simulink model "Linear_Approximation"  (R2019a)
settings: Solver=FixedStepDiscrete  StartTime=0.0  StopTime=t_end  RelTol=1e-3
InitFcn:
  | clear;
  | DIAGNOSTIC = 0;  %% flag to give more information as simulation proceeds such as comments & plots
  | CALIB_DIAGNOSTIC =  0; %% flag to give more information about calibration of filterbank due to overlap between filters: Mar 2016
  | PRESCRIPT = 1;  %% flag to plot requested versus achieved insertion gains (esp for 125-250 Hz region).
  | ipfiledigrms = -36; %% input file RMS in dB for 65 dB SPL equivalent
  | opfiledigrms = -36; %% output file RMS in dB for 65 dB SPL equivalent
  | equiv_ipSPL = 65; %% simulation of signal at this level through aid`
  | X_high = 1; % Maximum input
  | ref_dB = 85; X_ref = 1; % Define a reference point in X and its dBA value
  | re_level = 10.^(.05*(equiv_ipSPL-65)); %% scale factor at start of hearing aid, to get input to desired simulation level
  | M_bits = 5;   % decides length of tables, 2^(4+M_bits)
  | 
  | NChans = 5;
  | [chan_cfs, chan_thrs, t_atts, t_rels] ...
  |    = InitializeCompressionSettings(NChans);
  | % AidSettings5Chans;
  | 
  | %[VALID_WAV_FILE, sig, Fs, nbits, file_rms_dB, NStreams] ...
  | %  = loadwavfile(ipfiledigrms); %%  find [Fs], performs [recalculate] externally, provided valid file found
  | VALID_WAV_FILE = 1;
  | %[newfile, newpath] = uigetfile('*.wav','Open Signal File To Process.....');
  | %if isequal(newfile,0) || isequal(newpath,0)
  | %    fprintf(1,'\nFile not found'); VALID_WAV_FILE = 0;
  | %else
  | %    [sig, Fs] = audioread(strcat(newpath,newfile));
  | %end
  | X_thresh = 1*10^(0.05*(0-85));
  | 
  | Amplitudes = [X_thresh, X_thresh*10, X_thresh*100, X_thresh*1000, X_thresh*10000, 1]; %, X_thresh*100000];
  | 
  | fMin = 100; %Hz
  | fMax = 10000; %Hz
  | Fs = 48000; %Hz
  | Ts = 1/Fs;
  | %tt = (0:length(sig)-1 )./Fs;
  | tt = 0:Ts:4;
  | deltaF = (fMax - fMin)/tt(end);
  | X_sweep = Amplitudes'*sin(2*pi*(fMin*tt +  0.5*deltaF*tt.*tt)) ;
  | 
  | Fs = 48000;
  | Volume = 6;
  | sig = X_sweep(Volume,:)';
  | opplayer  = audioplayer(sig, Fs);
  | nbits = opplayer.bitspersample;
  | %sig = resample(sig,48000,Fs);
  | %Fs = 48000;
  | 
  | 
  | NStreams = min(size(sig));
  | EQ_SPAN_MSEC = 6;
  | 
  | insrt_frqs = [125, 250, 500, 1000, 2000, 3000, 4000, 6000, 8000, 10000 ]; %% decimal values
  | insrt_gns = [0 3 5 10 15 20 25 30 30 30]; %% prescribed dB for 65 dB input
  | %insrt_gns = 5*ones(1,length(insrt_frqs));  %no prescription
  | n_insrts = length(insrt_gns);
  | 
  | UPPER_FREQ_LIM = min(11e3, 0.90*Fs/2);
  | [ig_eq, calib_bpfs, dig_chan_lvl_0dBgain, dig_chan_dBthrs, Calib_recomb_dBpost] ...
  |     = update_channel_params(Fs, NChans, chan_cfs, chan_thrs, insrt_frqs, insrt_gns, ...
  |     0.1, UPPER_FREQ_LIM, EQ_SPAN_MSEC, PRESCRIPT, DIAGNOSTIC, CALIB_DIAGNOSTIC) ;  %% calculates channel edge frequencies, generates expected band levels for LTASS SWN to calibrate compressors & filterbank
  | 
  | recombGain = 10.^(0.05.*Calib_recomb_dBpost);
  | 
  | % translate sig into a form simulink likes
  | % Ts = 1/Fs;
  | % tt = (0:length(sig)-1).*Ts;
  | %t_end = tt(5*2^(M_bits+4) );   % to test table fill
  | t_end = tt(end);
  | sig_in = [tt', sig];
  | min_thresh_dB = 0;
  | for ix = 1:NChans
  |    [Gain_Table(:,ix), max_gain_prescript(ix), X_in(:,ix), chan_crs(ix)] ...
  |      = Compression_Wrapper_V2(Fs, min_thresh_dB, ...
  |      X_high, calib_bpfs(:,ix), ig_eq, ref_dB, X_ref, M_bits);
  | end
  | 
  | Initialize_Delay_Values;
  | Initialize_AGC_Consts;
  | W_bits = 32;
  | F_bits = 28;
  | M_bits = 5;
  | M_Bits = M_bits;
  | 
  | % Generating signals for simulink
  | Table_Fill = zeros(1,length(tt))';
  | Table_Fill(1                : 2^(M_bits+4) )  = Gain_Table(:,1);
  | Table_Fill(2^(M_bits+4)+1   : 2*2^(M_bits+4) )= Gain_Table(:,2);
  | Table_Fill(2*2^(M_bits+4)+1 : 3*2^(M_bits+4) )= Gain_Table(:,3);
  | Table_Fill(3*2^(M_bits+4)+1 : 4*2^(M_bits+4) )= Gain_Table(:,4);
  | Table_Fill(4*2^(M_bits+4)+1 : 5*2^(M_bits+4) )= Gain_Table(:,5);
  | Table_Fill = [tt', Table_Fill];
  | Fill_Valid = zeros(1,length(tt))';
  | Fill_Valid(1:5*2^(M_bits+4)) = 1;
  | Fill_Valid = boolean(Fill_Valid);
  | Fill_Valid = [tt', Fill_Valid];
  | t_att = t_atts./1000; s_att = t_att.*Fs; % change units of t_atts from ms to samples
  | t_rel = t_rels./1000; s_rel = t_rel.*Fs; % change units of t_rels from ms to samples
  | r_att = nthroot(0.1, s_att);
  | r_rel = nthroot(0.1, s_rel);
  | 
  | Reset = [tt', boolean(zeros(1,length(tt)))'];
StopFcn:
  | proc_sig = double(out.proc_sig.data(:));
  | %alignedSigs = double(out.alignedSigs.data(:));
  | [opwav, stop_ok] = savewavfile(opfiledigrms, ipfiledigrms, proc_sig, Fs, nbits, NStreams);
  | 
  | load('SweepSimOutput.mat')
  | X_out_Sweep_Sim(Volume,:) = proc_sig;
  | save('SweepSimOutput.mat', 'X_out_Sweep_Sim');
libraries: hdlsllib x33, simulink x2
settings Model: Creator=Bailey  LastModifiedBy=Bailey
settings DataIOCC: SaveOutput=off  SaveTime=off
settings OptimizationCC: BlockReduction=off  ConditionallyExecuteInputs=off  DefaultParameterBehavior=Inlined
settings DebuggingCC: AlgebraicLoopMsg=error  SingleTaskRateTransMsg=error
settings HardwareCC: ProdBitPerPointer=32  ProdBitPerSizeT=32  ProdBitPerPtrDiffT=32  ProdLargestAtomicFloat=None  ProdIntDivRoundTo=Undefined  ProdEndianess=Unspecified  ProdWordSize=32  ProdHWDeviceType=ASIC/FPGA->ASIC/FPGA  TargetBitPerPointer=64  TargetBitPerSizeT=64  TargetBitPerPtrDiffT=64  TargetLongLongMode=on  TargetIntDivRoundTo=Zero  TargetEndianess=LittleEndian  TargetWordSize=64  TargetHWDeviceType=Custom Processor->MATLAB Host Computer  ProdEqTarget=off

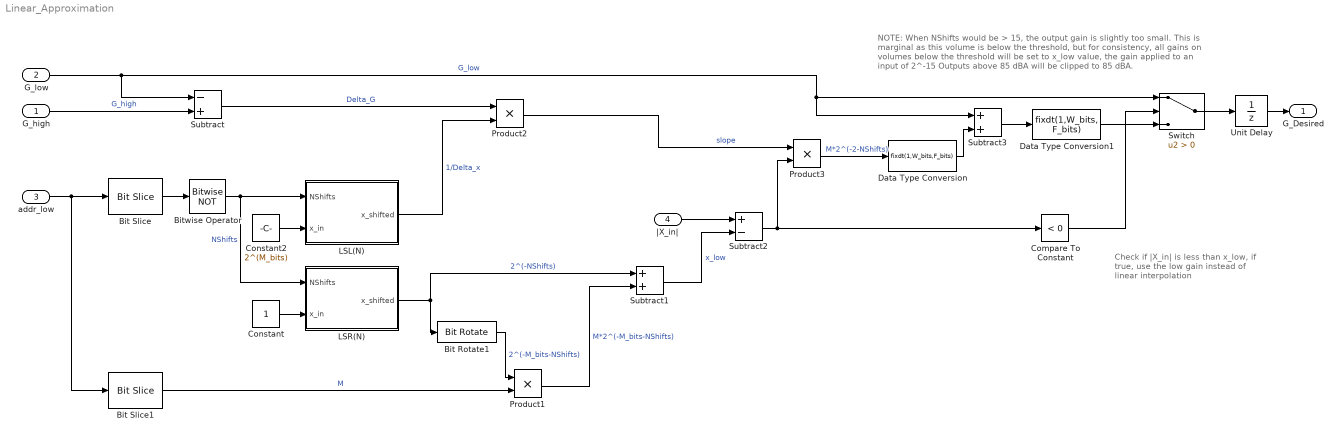
== system Linear_Approximation ==
  note: Check if |X_in| is less than x_low,
      | if true, use the low gain instead of
      | linear interpolation
  note: NOTE: When NShifts would be > 15, the output gain is slightly too small.
      | This is marginal as this volume is below the threshold, but for consistency,
      | all gains on volumes below the threshold will be set to x_low value, the
      | gain applied to an input of 2^-15
      | Outputs above 85 dBA will be clipped to 85 dBA.
  G_high : Inport  OutDataTypeStr=fixdt(1,32,28)  PortDimensions=1  SampleTime=[2.0833333333333333e-05,0]
  G_low : Inport  Port=2  OutDataTypeStr=fixdt(1,32,28)  PortDimensions=1  SampleTime=[2.0833333333333333e-05,0]
  addr_low : Inport  Port=3  OutDataTypeStr=fixdt(0,9,0)  PortDimensions=1  SampleTime=[2.0833333333333333e-05,0]
  |X_in| : Inport  Port=4  OutDataTypeStr=fixdt(1,32,28)  PortDimensions=1  SampleTime=[2.0833333333333333e-05,0]
  Bit Rotate1 : hdlsllib/Logic and Bit Operations/Bit Rotate  mode=Rotate Right  N=M_Bits
      settings: SourceProductName=Simulink  SourceProductBaseCode=SL
  Bit Slice : hdlsllib/Logic and Bit Operations/Bit Slice  lidx=M_Bits+3  ridx=M_Bits
      settings: SourceProductName=Simulink  SourceProductBaseCode=SL
  Bit Slice1 : hdlsllib/Logic and Bit Operations/Bit Slice  lidx=M_Bits-1  ridx=0
      settings: SourceProductName=Simulink  SourceProductBaseCode=SL
  Bitwise Operator : simulink/Logic and Bit Operations/Bitwise Operator  logicop=NOT  UseBitMask=off  BitMask=bin2dec('11011001')  BitMaskRealWorld=Stored Integer
  Compare To Constant : simulink/Logic and Bit Operations/Compare To Constant  relop=<  const=0  OutDataTypeStr=boolean
  Constant : Constant  OutDataTypeStr=fixdt(0,W_bits,W_bits-2)  SampleTime=-1
  Constant2 : Constant  Value=2^(M_bits)  OutDataTypeStr=fixdt(0,W_bits,0)  SampleTime=-1
  Data Type Conversion : DataTypeConversion  OutDataTypeStr=fixdt(1,W_bits,F_bits)
  Data Type Conversion1 : DataTypeConversion  OutDataTypeStr=fixdt(1,W_bits, F_bits)
  LSL(N) : Subsystem
  LSR(N) : Subsystem
  Product1 : Product
  Product2 : Product
  Product3 : Product
  Subtract : Sum  Inputs=-+
  Subtract1 : Sum  OutDataTypeStr=fixdt(1,W_bits, F_bits)
  Subtract2 : Sum  Inputs=+-  OutDataTypeStr=Inherit: Same as first input
  Subtract3 : Sum
  Switch : Switch  Criteria=u2 > Threshold
  Unit Delay : UnitDelay  InitialCondition=1  SampleTime=-1  HasFrameUpgradeWarning=on
  G_Desired : Outport  OutDataTypeStr=fixdt(1,32,28)  PortDimensions=1  SampleTime=[2.0833333333333333e-05,0]
  wires:
  addr_low/1 -> Bit Slice/1, Bit Slice1/1
  Bit Slice/1 -> Bitwise Operator/1
  Bitwise Operator/1 -> LSL(N)/1(NShifts), LSR(N)/1(NShifts)  "NShifts"
  Bit Slice1/1 -> Product1/2  "M"
  G_high/1 -> Subtract/2  "G_high"
  G_low/1 -> Subtract3/1, Switch/1, Subtract/1  "G_low"
  Subtract/1 -> Product2/1  "Delta_G"
  Constant/1 -> LSR(N)/2(x_in)
  LSR(N)/1(x_shifted) -> Subtract1/1, Bit Rotate1/1  "2^(-NShifts)"
  Bit Rotate1/1 -> Product1/1  "2^(-M_bits-NShifts)"
  Product1/1 -> Subtract1/2  "M*2^(-M_bits-NShifts)"
  Subtract1/1 -> Subtract2/2  "x_low"
  LSL(N)/1(x_shifted) -> Product2/2  "1/Delta_x"
  Product2/1 -> Product3/1  "slope"
  |X_in|/1 -> Subtract2/1
  Subtract2/1 -> Product3/2, Compare To Constant/1
  Product3/1 -> Data Type Conversion/1  "M*2^(-2-NShifts)"
  Subtract3/1 -> Data Type Conversion1/1
  Constant2/1 -> LSL(N)/2(x_in)
  Data Type Conversion/1 -> Subtract3/2
  Data Type Conversion1/1 -> Switch/3
  Unit Delay/1 -> G_Desired/1
  Compare To Constant/1 -> Switch/2
  Switch/1 -> Unit Delay/1

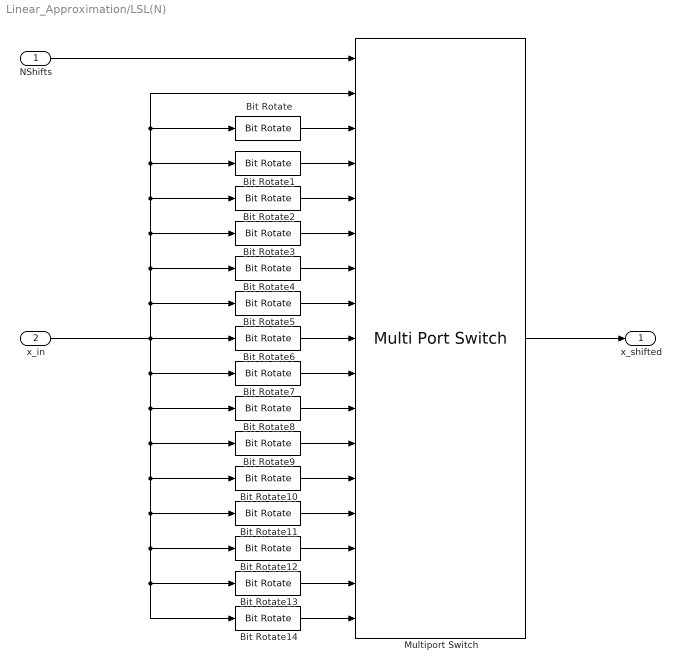
== system Linear_Approximation/LSL(N) ==
  NShifts : Inport
  x_in : Inport  Port=2
  Bit Rotate : hdlsllib/Logic and Bit Operations/Bit Rotate  mode=Rotate Left  N=1
      settings: SourceProductName=Simulink  SourceProductBaseCode=SL
  Bit Rotate1 : hdlsllib/Logic and Bit Operations/Bit Rotate  mode=Rotate Left  N=2
      settings: SourceProductName=Simulink  SourceProductBaseCode=SL
  Bit Rotate10 : hdlsllib/Logic and Bit Operations/Bit Rotate  mode=Rotate Left  N=11
      settings: SourceProductName=Simulink  SourceProductBaseCode=SL
  Bit Rotate11 : hdlsllib/Logic and Bit Operations/Bit Rotate  mode=Rotate Left  N=12
      settings: SourceProductName=Simulink  SourceProductBaseCode=SL
  Bit Rotate12 : hdlsllib/Logic and Bit Operations/Bit Rotate  mode=Rotate Left  N=13
      settings: SourceProductName=Simulink  SourceProductBaseCode=SL
  Bit Rotate13 : hdlsllib/Logic and Bit Operations/Bit Rotate  mode=Rotate Left  N=14
      settings: SourceProductName=Simulink  SourceProductBaseCode=SL
  Bit Rotate14 : hdlsllib/Logic and Bit Operations/Bit Rotate  mode=Rotate Left  N=15
      settings: SourceProductName=Simulink  SourceProductBaseCode=SL
  Bit Rotate2 : hdlsllib/Logic and Bit Operations/Bit Rotate  mode=Rotate Left  N=3
      settings: SourceProductName=Simulink  SourceProductBaseCode=SL
  Bit Rotate3 : hdlsllib/Logic and Bit Operations/Bit Rotate  mode=Rotate Left  N=4
      settings: SourceProductName=Simulink  SourceProductBaseCode=SL
  Bit Rotate4 : hdlsllib/Logic and Bit Operations/Bit Rotate  mode=Rotate Left  N=5
      settings: SourceProductName=Simulink  SourceProductBaseCode=SL
  Bit Rotate5 : hdlsllib/Logic and Bit Operations/Bit Rotate  mode=Rotate Left  N=6
      settings: SourceProductName=Simulink  SourceProductBaseCode=SL
  Bit Rotate6 : hdlsllib/Logic and Bit Operations/Bit Rotate  mode=Rotate Left  N=7
      settings: SourceProductName=Simulink  SourceProductBaseCode=SL
  Bit Rotate7 : hdlsllib/Logic and Bit Operations/Bit Rotate  mode=Rotate Left  N=8
      settings: SourceProductName=Simulink  SourceProductBaseCode=SL
  Bit Rotate8 : hdlsllib/Logic and Bit Operations/Bit Rotate  mode=Rotate Left  N=9
      settings: SourceProductName=Simulink  SourceProductBaseCode=SL
  Bit Rotate9 : hdlsllib/Logic and Bit Operations/Bit Rotate  mode=Rotate Left  N=10
      settings: SourceProductName=Simulink  SourceProductBaseCode=SL
  Multiport Switch : MultiPortSwitch  DataPortOrder=Zero-based contiguous  Inputs=16  DiagnosticForDefault=Warning  zeroidx=on
  x_shifted : Outport
  wires:
  Bit Rotate14/1 -> Multiport Switch/17
  Bit Rotate13/1 -> Multiport Switch/16
  Bit Rotate12/1 -> Multiport Switch/15
  Bit Rotate11/1 -> Multiport Switch/14
  Bit Rotate10/1 -> Multiport Switch/13
  Bit Rotate9/1 -> Multiport Switch/12
  Bit Rotate8/1 -> Multiport Switch/11
  Bit Rotate7/1 -> Multiport Switch/10
  Bit Rotate6/1 -> Multiport Switch/9
  Bit Rotate5/1 -> Multiport Switch/8
  Bit Rotate4/1 -> Multiport Switch/7
  Bit Rotate3/1 -> Multiport Switch/6
  Bit Rotate2/1 -> Multiport Switch/5
  Bit Rotate1/1 -> Multiport Switch/4
  Bit Rotate/1 -> Multiport Switch/3
  x_in/1 -> Bit Rotate6/1, Bit Rotate3/1, Bit Rotate2/1, Bit Rotate1/1, Bit Rotate/1, Multiport Switch/2, Bit Rotate4/1, Bit Rotate5/1, Bit Rotate7/1, Bit Rotate8/1, Bit Rotate9/1, Bit Rotate10/1, Bit Rotate11/1, Bit Rotate14/1, Bit Rotate13/1, Bit Rotate12/1
  Multiport Switch/1 -> x_shifted/1
  NShifts/1 -> Multiport Switch/1

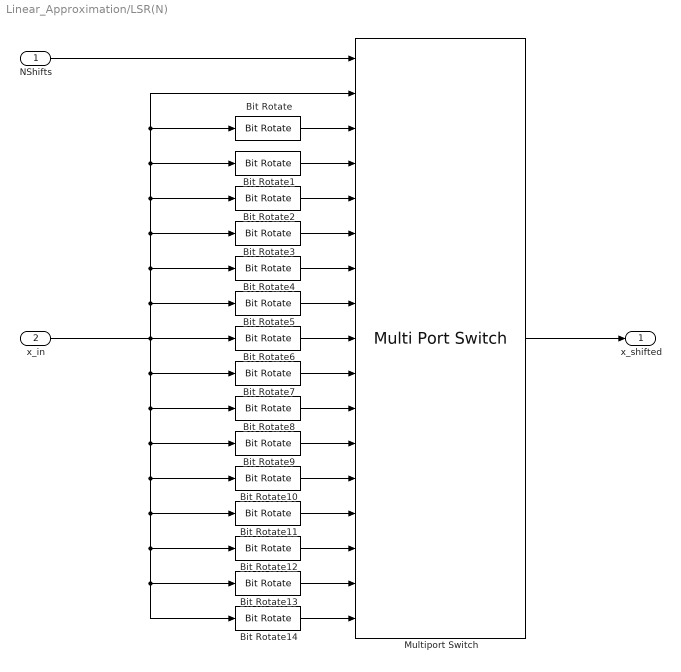
== system Linear_Approximation/LSR(N) ==
  NShifts : Inport
  x_in : Inport  Port=2
  Bit Rotate : hdlsllib/Logic and Bit Operations/Bit Rotate  mode=Rotate Right  N=1
      settings: SourceProductName=Simulink  SourceProductBaseCode=SL
  Bit Rotate1 : hdlsllib/Logic and Bit Operations/Bit Rotate  mode=Rotate Right  N=2
      settings: SourceProductName=Simulink  SourceProductBaseCode=SL
  Bit Rotate10 : hdlsllib/Logic and Bit Operations/Bit Rotate  mode=Rotate Right  N=11
      settings: SourceProductName=Simulink  SourceProductBaseCode=SL
  Bit Rotate11 : hdlsllib/Logic and Bit Operations/Bit Rotate  mode=Rotate Right  N=12
      settings: SourceProductName=Simulink  SourceProductBaseCode=SL
  Bit Rotate12 : hdlsllib/Logic and Bit Operations/Bit Rotate  mode=Rotate Right  N=13
      settings: SourceProductName=Simulink  SourceProductBaseCode=SL
  Bit Rotate13 : hdlsllib/Logic and Bit Operations/Bit Rotate  mode=Rotate Right  N=14
      settings: SourceProductName=Simulink  SourceProductBaseCode=SL
  Bit Rotate14 : hdlsllib/Logic and Bit Operations/Bit Rotate  mode=Rotate Right  N=15
      settings: SourceProductName=Simulink  SourceProductBaseCode=SL
  Bit Rotate2 : hdlsllib/Logic and Bit Operations/Bit Rotate  mode=Rotate Right  N=3
      settings: SourceProductName=Simulink  SourceProductBaseCode=SL
  Bit Rotate3 : hdlsllib/Logic and Bit Operations/Bit Rotate  mode=Rotate Right  N=4
      settings: SourceProductName=Simulink  SourceProductBaseCode=SL
  Bit Rotate4 : hdlsllib/Logic and Bit Operations/Bit Rotate  mode=Rotate Right  N=5
      settings: SourceProductName=Simulink  SourceProductBaseCode=SL
  Bit Rotate5 : hdlsllib/Logic and Bit Operations/Bit Rotate  mode=Rotate Right  N=6
      settings: SourceProductName=Simulink  SourceProductBaseCode=SL
  Bit Rotate6 : hdlsllib/Logic and Bit Operations/Bit Rotate  mode=Rotate Right  N=7
      settings: SourceProductName=Simulink  SourceProductBaseCode=SL
  Bit Rotate7 : hdlsllib/Logic and Bit Operations/Bit Rotate  mode=Rotate Right  N=8
      settings: SourceProductName=Simulink  SourceProductBaseCode=SL
  Bit Rotate8 : hdlsllib/Logic and Bit Operations/Bit Rotate  mode=Rotate Right  N=9
      settings: SourceProductName=Simulink  SourceProductBaseCode=SL
  Bit Rotate9 : hdlsllib/Logic and Bit Operations/Bit Rotate  mode=Rotate Right  N=10
      settings: SourceProductName=Simulink  SourceProductBaseCode=SL
  Multiport Switch : MultiPortSwitch  DataPortOrder=Zero-based contiguous  Inputs=16  DiagnosticForDefault=Warning  zeroidx=on
  x_shifted : Outport
  wires:
  Bit Rotate14/1 -> Multiport Switch/17
  Bit Rotate13/1 -> Multiport Switch/16
  Bit Rotate12/1 -> Multiport Switch/15
  Bit Rotate11/1 -> Multiport Switch/14
  Bit Rotate10/1 -> Multiport Switch/13
  Bit Rotate9/1 -> Multiport Switch/12
  Bit Rotate8/1 -> Multiport Switch/11
  Bit Rotate7/1 -> Multiport Switch/10
  Bit Rotate6/1 -> Multiport Switch/9
  Bit Rotate5/1 -> Multiport Switch/8
  Bit Rotate4/1 -> Multiport Switch/7
  Bit Rotate3/1 -> Multiport Switch/6
  Bit Rotate2/1 -> Multiport Switch/5
  Bit Rotate1/1 -> Multiport Switch/4
  Bit Rotate/1 -> Multiport Switch/3
  x_in/1 -> Bit Rotate6/1, Bit Rotate3/1, Bit Rotate2/1, Bit Rotate1/1, Bit Rotate/1, Multiport Switch/2, Bit Rotate4/1, Bit Rotate5/1, Bit Rotate7/1, Bit Rotate8/1, Bit Rotate9/1, Bit Rotate10/1, Bit Rotate11/1, Bit Rotate14/1, Bit Rotate13/1, Bit Rotate12/1
  Multiport Switch/1 -> x_shifted/1
  NShifts/1 -> Multiport Switch/1
